simulink model "sumulacionTpBolita"  (R2019b)
settings: Solver=ode4  StartTime=0.0  StopTime=5  FixedStep=10e-6  RelTol=1e-3
undefined symbols (not defined in the file or in its folder): A0, Acd, Aoc, B0, Bcd, Boc, c, C0, Ccd, Coc, Dcd, DiscIntNeverNeededParam, Doc, K, Ki, L, Pade, Tsample, u0, x0, x0f
libraries: cstblocks x2
settings Model: Creator=mpier  LastModifiedBy=mpier
settings ConfigComp: PLC_TargetIDE=codesys23

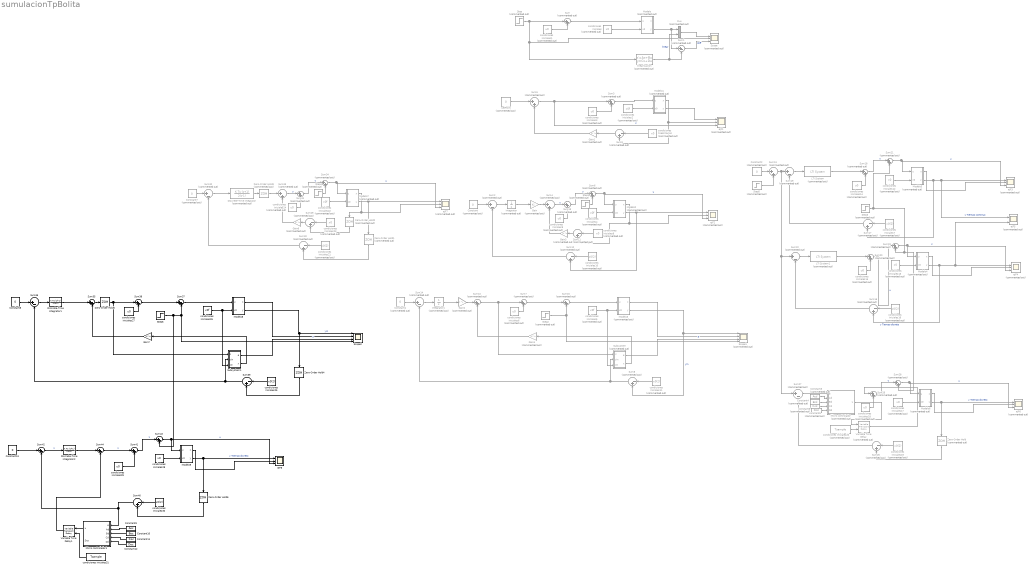
== system sumulacionTpBolita ==
  " Micro controlador" : MATLAB Function  Commented=on  TreatAsAtomicUnit=on  SystemSampleTime=Tsample
  " Micro controlador1" : MATLAB Function  TreatAsAtomicUnit=on  SystemSampleTime=Tsample
  Constant{,1..2,7} (4 alike) : Constant  Commented=on  Value=0
  Constant10 : Constant  Value=Boc
  Constant11 : Constant  Value=Coc
  Constant12 : Constant  Value=Doc
  Constant13 : Constant  Value=0
  Constant3 : Constant  Commented=on  Value=Acd
  Constant4 : Constant  Commented=on  Value=Bcd
  Constant5 : Constant  Commented=on  Value=Ccd
  Constant6 : Constant  Commented=on  Value=Dcd
  Constant8 : Constant  Value=0
  Constant9 : Constant  Value=Aoc
  Discrete-Time Integrator : DiscreteIntegrator  Commented=on  IntegratorMethod=Integration: Trapezoidal  gainval=Ki  SampleTime=Tsample  ICPrevOutput=DiscIntNeverNeededParam  ICPrevScaledInput=DiscIntNeverNeededParam
  Discrete-Time Integrator1 : DiscreteIntegrator  IntegratorMethod=Integration: Trapezoidal  gainval=Ki  SampleTime=Tsample  ICPrevOutput=DiscIntNeverNeededParam  ICPrevScaledInput=DiscIntNeverNeededParam
  Discrete-Time Integrator2 : DiscreteIntegrator  IntegratorMethod=Integration: Trapezoidal  gainval=Ki  SampleTime=Tsample  ICPrevOutput=DiscIntNeverNeededParam  ICPrevScaledInput=DiscIntNeverNeededParam
  Gain : Gain  Commented=on  Gain=Ki
  Gain{1,3..4,6} (4 alike) : Gain  Commented=on  Gain=-K  Multiplication=Matrix(K*u)
  Gain2 : Gain  Commented=on  Gain=Ki  Multiplication=Matrix(K*u)
  Gain7 : Gain  Gain=-K  Multiplication=Matrix(K*u)
  Integrator : Integrator  Commented=on
  Integrator1 : Integrator  Commented=on
  LTI System : cstblocks/LTI System  Commented=on  sys=c*Pade  IC=[]
  LTI System1 : cstblocks/LTI System  Commented=on  sys=Cd  IC=[]
  Modelo : Subsystem  Commented=on
  Modelo1 : Subsystem  Commented=on
  Modelo2 : Subsystem  Commented=on
  Modelo3 : Subsystem  Commented=on
  Modelo4 : Subsystem  Commented=on
  Modelo5 : Subsystem  Commented=on
  Modelo6 : Subsystem  Commented=on
  Modelo7 : Subsystem  Commented=on
  Modelo8 : Subsystem
  Modelo9 : Subsystem
  Mux : Mux  Commented=on  Inputs=2
  Scope : Scope  Commented=on  NumInputPorts=3
  Scope1 : Scope  Commented=on  NumInputPorts=4
  Scope2 : Scope  NumInputPorts=4
  Step : Step  Commented=on  Time=50e-3  After=0.1  SampleTime=0
  Step1 : Step  Commented=on  Time=2.5  After=10  SampleTime=0
  Step2 : Step  Commented=on  Time=2.5  After=2  SampleTime=0
  Step3 : Step  Commented=on  Time=2.5  After=100e-3  SampleTime=0
  Step4 : Step  Commented=on  Time=2.5  After=10  SampleTime=0
  Step5 : Step  Commented=on  After=1e-3  SampleTime=0
  Step6 : Step  Time=2.5  After=1e-3  SampleTime=0
  Subsystem : Subsystem  Commented=on
  Subsystem1 : Subsystem
  Sum{,3,6..7,10,13,15,18,20..21,23,26,28,31,34} (15 alike) : Sum  Commented=on  Inputs=|++
  Sum1 : Sum  Commented=on  Inputs=|+-
  Sum{8..9,11..12,16..17,25,29..30} (9 alike) : Sum  Commented=on  Inputs=|-+  OutDataTypeStr=double
  Sum{2,14,19,22,27,32} (6 alike) : Sum  Commented=on  Inputs=|+-  OutDataTypeStr=double
  Sum{4..5,24,33} (4 alike) : Sum  Commented=on  Inputs=|++  OutDataTypeStr=double
  Sum{35,37..38,41,43} (5 alike) : Sum  Inputs=|++
  Sum36 : Sum  Inputs=|+-  OutDataTypeStr=double
  Sum39 : Sum  Inputs=|-+  OutDataTypeStr=double
  Sum40 : Sum  Inputs=|-+  OutDataTypeStr=double
  Sum42 : Sum  Inputs=|+-
  Sum44 : Sum  Inputs=|+-
  Variable Time Delay : VariableTransportDelay  Commented=on  MaximumDelay=10
  Variable Time Delay1 : VariableTransportDelay  MaximumDelay=10
  Zero-Order Hold : ZeroOrderHold  Commented=on  SampleTime=Tsample
  Zero-Order Hold1 : ZeroOrderHold  Commented=on  SampleTime=-1
  Zero-Order Hold2 : ZeroOrderHold  Commented=on  SampleTime=-1
  Zero-Order Hold3 : ZeroOrderHold  Commented=on  SampleTime=-1
  Zero-Order Hold4 : ZeroOrderHold  SampleTime=-1
  Zero-Order Hold5 : ZeroOrderHold  SampleTime=-1
  Zero-Order Hold6 : ZeroOrderHold  SampleTime=Tsample
  condiciones Iniciales{,8,12..13,17,23} (6 alike) : Constant  Commented=on  Value=x0
  condiciones Iniciales{1,3,6,9,14..15,18,24} (8 alike) : Constant  Commented=on  Value=u0
  condiciones Iniciales{7,10..11,16,19,21} (6 alike) : Constant  Commented=on  Value=x0(2)
  condiciones Iniciales{2,4..5,22} (4 alike) : Constant  Commented=on  Value=x0f
  condiciones Iniciales20 : Constant  Commented=on  Value=Tsample
  condiciones Iniciales25 : Constant  Value=x0(2)
  condiciones Iniciales26 : Constant  Value=x0f
  condiciones Iniciales27 : Constant  Value=u0
  condiciones Iniciales28 : Constant  Value=x0
  condiciones Iniciales29 : Constant  Value=u0
  condiciones Iniciales30 : Constant  Value=x0(2)
  condiciones Iniciales31 : Constant  Value=Tsample
  condiciones linealizacion : Constant  Commented=on  Value=x0
  ejF{1..4,6..7} (6 alike) : Scope  Commented=on  NumInputPorts=3
  ejF5 : Scope  Commented=on  NumInputPorts=2
  ejF8 : Scope  NumInputPorts=3
  linearizacion : StateSpace  Commented=on  A=A0  B=B0  C=C0  D=0  InitialCondition=0
  setPoint : Constant  Commented=on  Value=0
  wires:
  condiciones Iniciales/1 -> Modelo/2(x0)
  Sum/1 -> Modelo/1(u)
  condiciones Iniciales1/1 -> Sum/2
  Mux/1 -> Scope/1
  Modelo/2(y) -> Sum1/1, Mux/1
  linearizacion/1 -> Sum1/2, Mux/2  "linear"
  Sum1/1 -> Scope/3  "Diff"
  Step/1 -> linearizacion/1, Scope/2, Sum/1
  Modelo1/1(x) -> Sum9/2, ejF1/2
  condiciones Iniciales3/1 -> Sum3/2
  Sum3/1 -> Modelo1/1(u)
  condiciones Iniciales2/1 -> Modelo1/2(x0)
  Modelo1/2(y) -> ejF1/1
  Sum5/1 -> ejF1/3, Sum3/1  "u"
  Gain1/1 -> Sum5/2
  Modelo2/1(x) -> ejF2/2, Sum11/2
  condiciones Iniciales4/1 -> Modelo2/2(x0)
  Constant/1 -> Sum2/1
  Sum2/1 -> Integrator/1
  Integrator/1 -> Gain/1
  Gain/1 -> Sum4/1
  condiciones Iniciales5/1 -> Subsystem/3(x0), Modelo3/2(x0)
  Sum10/1 -> Sum7/1, Subsystem/1(u)
  Gain4/1 -> Sum10/2
  Sum9/1 -> Gain1/1
  condiciones linealizacion/1 -> Sum9/1
  setPoint/1 -> Sum5/1
  Sum11/1 -> Gain3/1
  condiciones Iniciales8/1 -> Sum11/1
  Gain3/1 -> Sum4/2
  Sum12/1 -> Sum2/2
  condiciones Iniciales9/1 -> Sum13/2
  Sum4/1 -> Sum13/1  "u"
  condiciones Iniciales10/1 -> Sum12/1
  condiciones Iniciales11/1 -> Sum8/1
  Subsystem/2(x) -> Gain4/1
  condiciones Iniciales6/1 -> Sum7/2
  Sum8/1 -> Sum14/2, Subsystem/2(yin)
  Gain2/1 -> Sum10/1
  Integrator1/1 -> Gain2/1
  Constant1/1 -> Sum14/1
  Sum14/1 -> Integrator1/1
  Modelo3/2(y) -> Sum8/2, Scope1/1  "yin"
  Modelo3/1(x) -> Scope1/2
  Subsystem/1(e) -> Scope1/3  "e"
  Modelo2/2(y) -> ejF2/1, Sum12/2
  Step1/1 -> Sum6/2
  Sum13/1 -> Sum6/1  "u"
  Sum6/1 -> ejF2/3, Modelo2/1(u)  "u"
  Sum7/1 -> Sum15/1
  Step2/1 -> Sum15/2, Scope1/4
  Sum15/1 -> Modelo3/1(u)
  condiciones Iniciales14/1 -> Sum18/2
  Modelo5/2(y) -> ejF5/1, ejF3/1, Sum17/2  "y Tiempo continuo"
  Sum19/1 -> LTI System/1
  Sum18/1 -> Sum21/1  "u"
  Sum17/1 -> Sum19/2
  Modelo5/1(x) -> ejF3/2
  Sum21/1 -> ejF3/3, Modelo5/1(u)  "u"
  condiciones Iniciales7/1 -> Sum17/1
  condiciones Iniciales12/1 -> Modelo5/2(x0)
  LTI System/1 -> Sum18/1
  condiciones Iniciales16/1 -> Sum16/1
  Sum23/1 -> ejF4/3, Modelo4/1(u)  "u"
  Sum16/1 -> Sum22/2
  Sum20/1 -> Sum23/1  "u"
  Modelo4/1(x) -> ejF4/2
  Sum22/1 -> LTI System1/1
  condiciones Iniciales15/1 -> Sum20/2
  Modelo4/2(y) -> ejF5/2, ejF4/1, Sum16/2  "y Tiempo dicreto"
  condiciones Iniciales13/1 -> Modelo4/2(x0)
  LTI System1/1 -> Sum20/1
  Constant2/1 -> Sum24/1
  Step5/1 -> Sum24/2
  Step3/1 -> Sum28/2, Sum23/2, Sum21/2
  condiciones Iniciales19/1 -> Sum25/1
  condiciones Iniciales18/1 -> Sum26/2
  Sum27/1 -> " Micro controlador"/1(e)
  Sum24/1 -> Sum19/1, Sum27/1, Sum22/1
  Sum28/1 -> ejF6/3, Modelo6/1(u)  "u"
  Sum26/1 -> Sum28/1  "u"
  Modelo6/1(x) -> ejF6/2
  condiciones Iniciales17/1 -> Modelo6/2(x0)
  Modelo6/2(y) -> ejF6/1, Zero-Order Hold/1  "y Tiempo dicreto"
  Sum25/1 -> Sum27/2
  Constant3/1 -> " Micro controlador"/2(Ad)
  Constant4/1 -> " Micro controlador"/3(Bd)
  Constant5/1 -> " Micro controlador"/4(Cd)
  Constant6/1 -> " Micro controlador"/5(Dd)
  " Micro controlador"/1(u) -> Variable Time Delay/1
  Variable Time Delay/1 -> Sum26/1
  condiciones Iniciales20/1 -> Variable Time Delay/2
  Zero-Order Hold/1 -> Sum25/2
  Modelo7/1(x) -> ejF7/2, Zero-Order Hold2/1
  Sum33/1 -> Sum31/1  "u"
  condiciones Iniciales23/1 -> Sum29/1
  Sum31/1 -> Sum34/1  "u"
  Modelo7/2(y) -> ejF7/1, Zero-Order Hold1/1
  Gain6/1 -> Sum33/2
  Sum32/1 -> Discrete-Time Integrator/1
  Step4/1 -> Sum34/2
  Discrete-Time Integrator/1 -> Zero-Order Hold3/1
  Sum34/1 -> ejF7/3, Modelo7/1(u)  "u"
  condiciones Iniciales21/1 -> Sum30/1
  Sum30/1 -> Sum32/2
  Sum29/1 -> Gain6/1
  condiciones Iniciales24/1 -> Sum31/2
  condiciones Iniciales22/1 -> Modelo7/2(x0)
  Constant7/1 -> Sum32/1
  Zero-Order Hold1/1 -> Sum30/2
  Zero-Order Hold2/1 -> Sum29/2
  Zero-Order Hold3/1 -> Sum33/1
  Sum36/1 -> Discrete-Time Integrator1/1
  Modelo8/2(y) -> Zero-Order Hold4/1, Scope2/1  "yin"
  Sum37/1 -> Modelo8/1(u)
  Modelo8/1(x) -> Scope2/2
  Sum35/1 -> Zero-Order Hold5/1
  condiciones Iniciales25/1 -> Sum39/1
  Sum38/1 -> Sum37/1
  Subsystem1/2(x) -> Gain7/1
  condiciones Iniciales27/1 -> Sum38/2
  condiciones Iniciales26/1 -> Subsystem1/3(x0), Modelo8/2(x0)
  Gain7/1 -> Sum35/2
  Discrete-Time Integrator1/1 -> Sum35/1
  Subsystem1/1(e) -> Scope2/3  "e"
  Sum39/1 -> Sum36/2, Subsystem1/2(yin)
  Zero-Order Hold4/1 -> Sum39/2
  Zero-Order Hold5/1 -> Subsystem1/1(u), Sum38/1
  condiciones Iniciales31/1 -> Variable Time Delay1/2
  Constant11/1 -> " Micro controlador1"/4(Cd)
  Constant10/1 -> " Micro controlador1"/3(Bd)
  condiciones Iniciales29/1 -> Sum41/2
  Sum43/1 -> ejF8/3, Modelo9/1(u)  "u"
  Modelo9/1(x) -> ejF8/2
  Zero-Order Hold6/1 -> Sum40/2
  Sum41/1 -> Sum43/1  "u"
  Constant12/1 -> " Micro controlador1"/5(Dd)
  Constant9/1 -> " Micro controlador1"/2(Ad)
  condiciones Iniciales28/1 -> Modelo9/2(x0)
  Constant8/1 -> Sum36/1
  condiciones Iniciales30/1 -> Sum40/1
  Step6/1 -> Sum43/2, Sum37/2, Scope2/4
  Modelo9/2(y) -> ejF8/1, Zero-Order Hold6/1  "y Tiempo dicreto"
  " Micro controlador1"/1(u) -> Variable Time Delay1/1
  Sum42/1 -> Discrete-Time Integrator2/1  "u"
  Sum40/1 -> Sum42/2, " Micro controlador1"/1(e)
  Sum44/1 -> Sum41/1  "u"
  Discrete-Time Integrator2/1 -> Sum44/1
  Variable Time Delay1/1 -> Sum44/2
  Constant13/1 -> Sum42/1

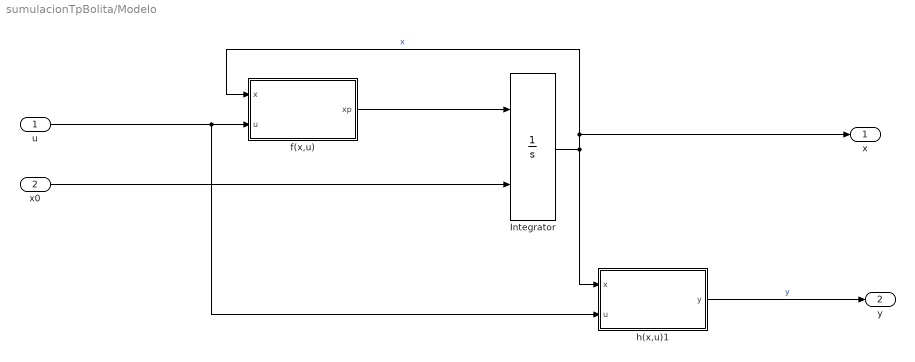
== system sumulacionTpBolita/Modelo ==
  u : Inport
  x0 : Inport  Port=2
  Integrator : Integrator  InitialConditionSource=external
  f(x,u) : MATLAB Function  TreatAsAtomicUnit=on
  h(x,u)1 : MATLAB Function  TreatAsAtomicUnit=on
  x : Outport
  y : Outport  Port=2
  wires:
  Integrator/1 -> x/1, f(x,u)/1(x), h(x,u)1/1(x)  "x"
  f(x,u)/1(xp) -> Integrator/1
  x0/1 -> Integrator/2
  u/1 -> h(x,u)1/2(u), f(x,u)/2(u)
  h(x,u)1/1(y) -> y/1  "y"

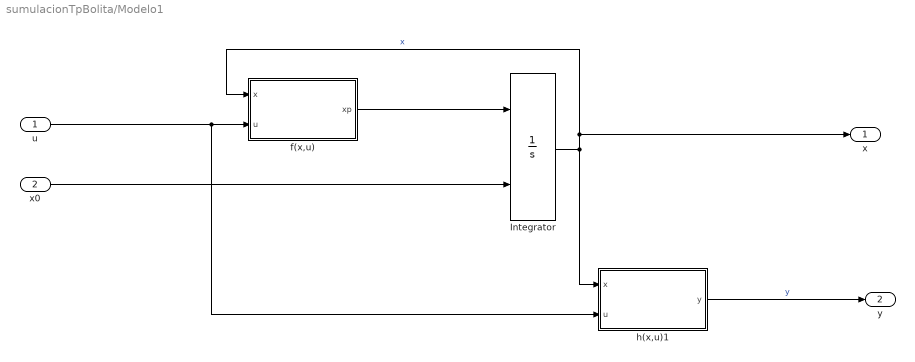
== system sumulacionTpBolita/Modelo1 ==
  u : Inport
  x0 : Inport  Port=2
  Integrator : Integrator  InitialConditionSource=external
  f(x,u) : MATLAB Function  TreatAsAtomicUnit=on
  h(x,u)1 : MATLAB Function  TreatAsAtomicUnit=on
  x : Outport
  y : Outport  Port=2
  wires:
  Integrator/1 -> x/1, f(x,u)/1(x), h(x,u)1/1(x)  "x"
  f(x,u)/1(xp) -> Integrator/1
  x0/1 -> Integrator/2
  u/1 -> h(x,u)1/2(u), f(x,u)/2(u)
  h(x,u)1/1(y) -> y/1  "y"

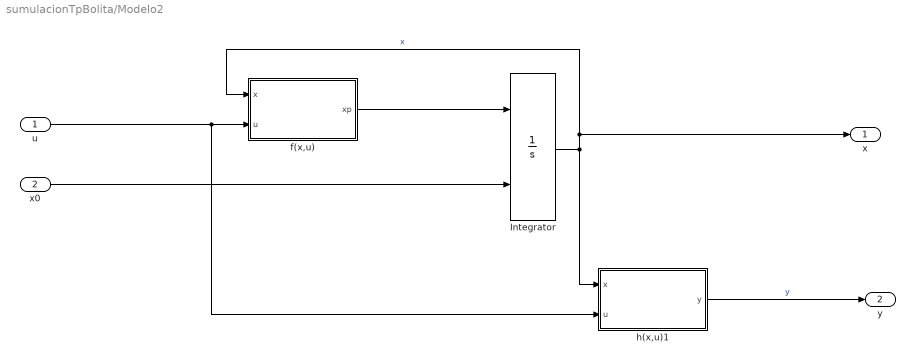
== system sumulacionTpBolita/Modelo2 ==
  u : Inport
  x0 : Inport  Port=2
  Integrator : Integrator  InitialConditionSource=external
  f(x,u) : MATLAB Function  TreatAsAtomicUnit=on
  h(x,u)1 : MATLAB Function  TreatAsAtomicUnit=on
  x : Outport
  y : Outport  Port=2
  wires:
  Integrator/1 -> x/1, f(x,u)/1(x), h(x,u)1/1(x)  "x"
  f(x,u)/1(xp) -> Integrator/1
  x0/1 -> Integrator/2
  u/1 -> h(x,u)1/2(u), f(x,u)/2(u)
  h(x,u)1/1(y) -> y/1  "y"

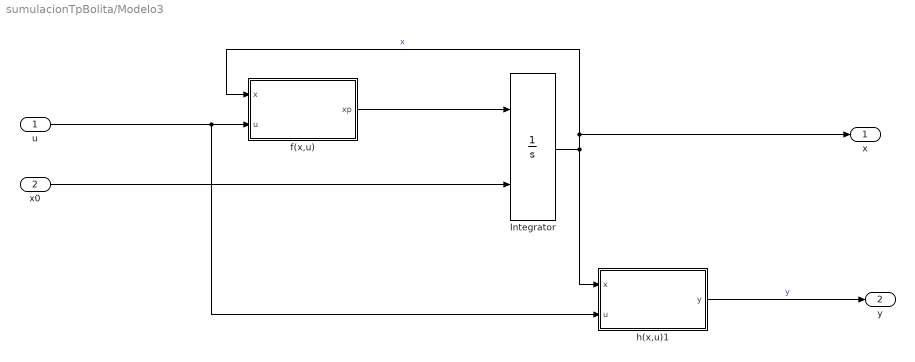
== system sumulacionTpBolita/Modelo3 ==
  u : Inport
  x0 : Inport  Port=2
  Integrator : Integrator  InitialConditionSource=external
  f(x,u) : MATLAB Function  TreatAsAtomicUnit=on
  h(x,u)1 : MATLAB Function  TreatAsAtomicUnit=on
  x : Outport
  y : Outport  Port=2
  wires:
  Integrator/1 -> x/1, f(x,u)/1(x), h(x,u)1/1(x)  "x"
  f(x,u)/1(xp) -> Integrator/1
  x0/1 -> Integrator/2
  u/1 -> h(x,u)1/2(u), f(x,u)/2(u)
  h(x,u)1/1(y) -> y/1  "y"

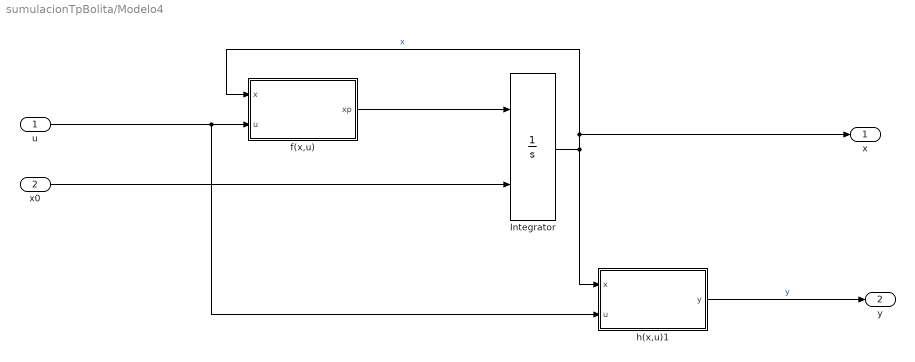
== system sumulacionTpBolita/Modelo4 ==
  u : Inport
  x0 : Inport  Port=2
  Integrator : Integrator  InitialConditionSource=external
  f(x,u) : MATLAB Function  TreatAsAtomicUnit=on
  h(x,u)1 : MATLAB Function  TreatAsAtomicUnit=on
  x : Outport
  y : Outport  Port=2
  wires:
  Integrator/1 -> x/1, f(x,u)/1(x), h(x,u)1/1(x)  "x"
  f(x,u)/1(xp) -> Integrator/1
  x0/1 -> Integrator/2
  u/1 -> h(x,u)1/2(u), f(x,u)/2(u)
  h(x,u)1/1(y) -> y/1  "y"

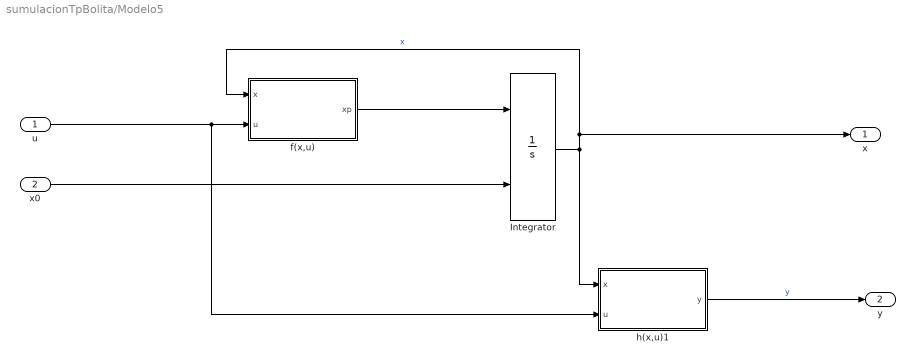
== system sumulacionTpBolita/Modelo5 ==
  u : Inport
  x0 : Inport  Port=2
  Integrator : Integrator  InitialConditionSource=external
  f(x,u) : MATLAB Function  TreatAsAtomicUnit=on
  h(x,u)1 : MATLAB Function  TreatAsAtomicUnit=on
  x : Outport
  y : Outport  Port=2
  wires:
  Integrator/1 -> x/1, f(x,u)/1(x), h(x,u)1/1(x)  "x"
  f(x,u)/1(xp) -> Integrator/1
  x0/1 -> Integrator/2
  u/1 -> h(x,u)1/2(u), f(x,u)/2(u)
  h(x,u)1/1(y) -> y/1  "y"

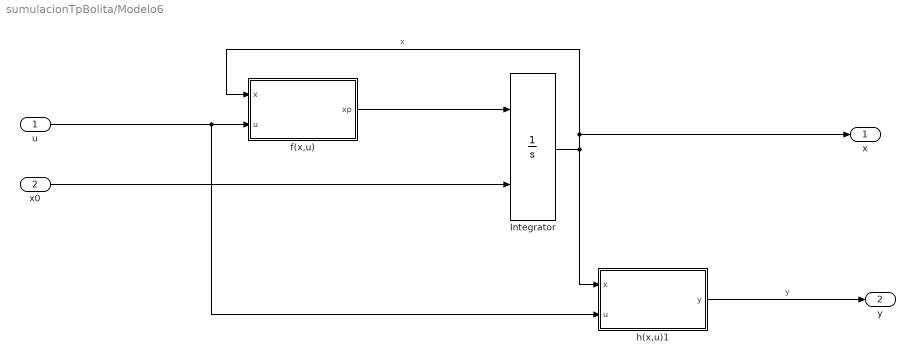
== system sumulacionTpBolita/Modelo6 ==
  u : Inport
  x0 : Inport  Port=2
  Integrator : Integrator  InitialConditionSource=external
  f(x,u) : MATLAB Function  TreatAsAtomicUnit=on
  h(x,u)1 : MATLAB Function  TreatAsAtomicUnit=on
  x : Outport
  y : Outport  Port=2
  wires:
  Integrator/1 -> x/1, f(x,u)/1(x), h(x,u)1/1(x)  "x"
  f(x,u)/1(xp) -> Integrator/1
  x0/1 -> Integrator/2
  u/1 -> h(x,u)1/2(u), f(x,u)/2(u)
  h(x,u)1/1(y) -> y/1  "y"

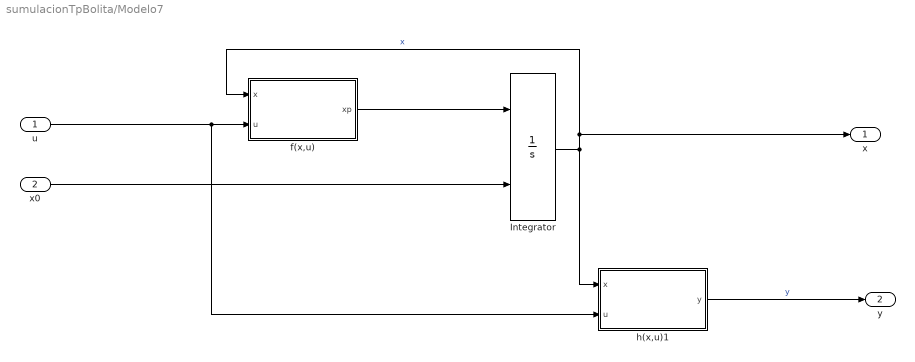
== system sumulacionTpBolita/Modelo7 ==
  u : Inport
  x0 : Inport  Port=2
  Integrator : Integrator  InitialConditionSource=external
  f(x,u) : MATLAB Function  TreatAsAtomicUnit=on
  h(x,u)1 : MATLAB Function  TreatAsAtomicUnit=on
  x : Outport
  y : Outport  Port=2
  wires:
  Integrator/1 -> x/1, f(x,u)/1(x), h(x,u)1/1(x)  "x"
  f(x,u)/1(xp) -> Integrator/1
  x0/1 -> Integrator/2
  u/1 -> h(x,u)1/2(u), f(x,u)/2(u)
  h(x,u)1/1(y) -> y/1  "y"

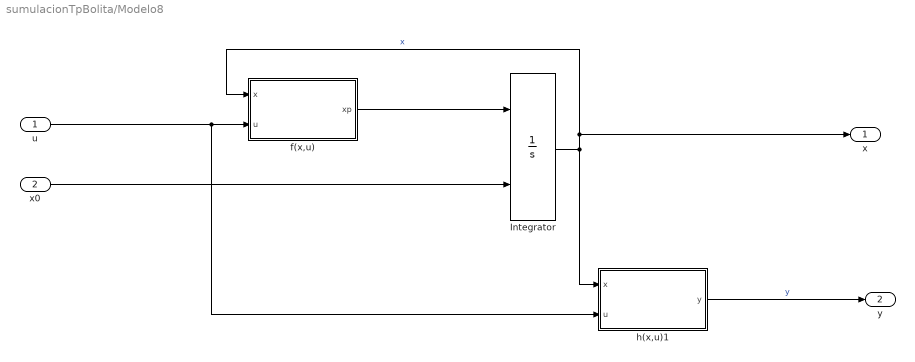
== system sumulacionTpBolita/Modelo8 ==
  u : Inport
  x0 : Inport  Port=2
  Integrator : Integrator  InitialConditionSource=external
  f(x,u) : MATLAB Function  TreatAsAtomicUnit=on
  h(x,u)1 : MATLAB Function  TreatAsAtomicUnit=on
  x : Outport
  y : Outport  Port=2
  wires:
  Integrator/1 -> x/1, f(x,u)/1(x), h(x,u)1/1(x)  "x"
  f(x,u)/1(xp) -> Integrator/1
  x0/1 -> Integrator/2
  u/1 -> h(x,u)1/2(u), f(x,u)/2(u)
  h(x,u)1/1(y) -> y/1  "y"

== system sumulacionTpBolita/Modelo9 ==
  u : Inport
  x0 : Inport  Port=2
  Integrator : Integrator  InitialConditionSource=external
  f(x,u) : MATLAB Function  TreatAsAtomicUnit=on
  h(x,u)1 : MATLAB Function  TreatAsAtomicUnit=on
  x : Outport
  y : Outport  Port=2
  wires:
  Integrator/1 -> x/1, f(x,u)/1(x), h(x,u)1/1(x)  "x"
  f(x,u)/1(xp) -> Integrator/1
  x0/1 -> Integrator/2
  u/1 -> h(x,u)1/2(u), f(x,u)/2(u)
  h(x,u)1/1(y) -> y/1  "y"

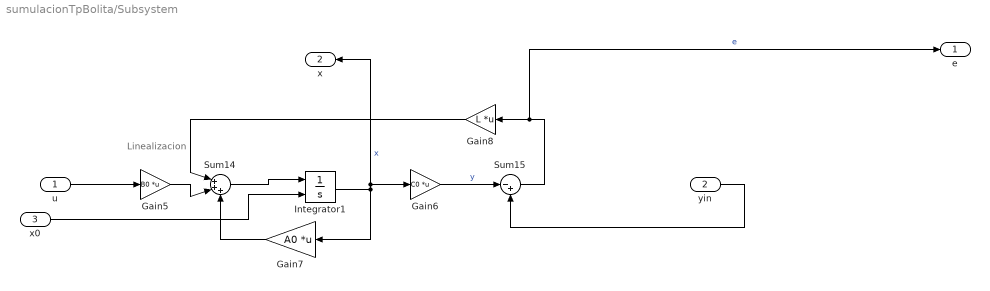
== system sumulacionTpBolita/Subsystem ==
  note: Linealizacion
  u : Inport
  yin : Inport  Port=2
  x0 : Inport  Port=3
  Gain5 : Gain  Gain=B0  Multiplication=Matrix(K*u)
  Gain6 : Gain  Gain=C0  Multiplication=Matrix(K*u)
  Gain7 : Gain  Gain=A0  Multiplication=Matrix(K*u)
  Gain8 : Gain  Gain=L  Multiplication=Matrix(K*u)
  Integrator1 : Integrator  InitialConditionSource=external
  Sum14 : Sum  Inputs=|+++
  Sum15 : Sum  Inputs=|-+
  e : Outport
  x : Outport  Port=2
  wires:
  u/1 -> Gain5/1
  Sum14/1 -> Integrator1/1
  yin/1 -> Sum15/2
  Integrator1/1 -> x/1, Gain6/1, Gain7/1  "x"
  Gain7/1 -> Sum14/3
  Sum15/1 -> e/1, Gain8/1  "e"
  Gain6/1 -> Sum15/1  "y"
  Gain5/1 -> Sum14/2
  Gain8/1 -> Sum14/1
  x0/1 -> Integrator1/2

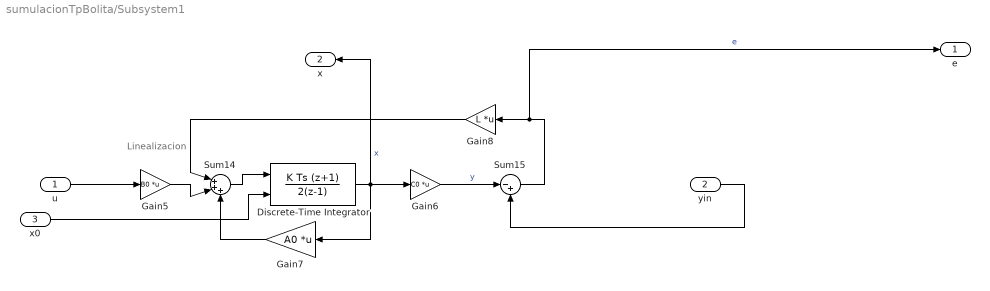
== system sumulacionTpBolita/Subsystem1 ==
  note: Linealizacion
  u : Inport
  yin : Inport  Port=2
  x0 : Inport  Port=3
  Discrete-Time Integrator : DiscreteIntegrator  IntegratorMethod=Integration: Trapezoidal  InitialConditionSource=external  SampleTime=Tsample  ICPrevOutput=DiscIntNeverNeededParam  ICPrevScaledInput=DiscIntNeverNeededParam
  Gain5 : Gain  Gain=B0  Multiplication=Matrix(K*u)
  Gain6 : Gain  Gain=C0  Multiplication=Matrix(K*u)
  Gain7 : Gain  Gain=A0  Multiplication=Matrix(K*u)
  Gain8 : Gain  Gain=L  Multiplication=Matrix(K*u)
  Sum14 : Sum  Inputs=|+++
  Sum15 : Sum  Inputs=|-+
  e : Outport
  x : Outport  Port=2
  wires:
  u/1 -> Gain5/1
  Sum14/1 -> Discrete-Time Integrator/1
  yin/1 -> Sum15/2
  Discrete-Time Integrator/1 -> x/1, Gain7/1, Gain6/1  "x"
  Gain7/1 -> Sum14/3
  Sum15/1 -> e/1, Gain8/1  "e"
  Gain6/1 -> Sum15/1  "y"
  Gain5/1 -> Sum14/2
  Gain8/1 -> Sum14/1
  x0/1 -> Discrete-Time Integrator/2

== matlab function sumulacionTpBolita/Modelo/h(x,u)1 ==
  data: x input; u input; y output
function y = h(x,u)



y=x(2);

== matlab function sumulacionTpBolita/Modelo/f(x,u) ==
  data: x input; u input; xp output
function xp = f(x,u)



R=4;%resistencia del inductor
 L=1;%inductancia del electro iman
 m=0.2;%masa de la bolita
 g=10;%aceleracion de la grabedad
 

ids=(-(x(1)^2)/(L/R))+(u/L);

F1s=(0.5*((2+x(1))^2))/((1-x(2))^2);
F2s=(0.5*((2-x(1))^2))/((1+x(2))^2);
vds=-g+(F1s/m)-(F2s/m);

xp=[ids;x(3);vds];

== matlab function sumulacionTpBolita/Modelo1/f(x,u) ==
  data: x input; u input; xp output
function xp = f(x,u)



R=4;%resistencia del inductor
 L=1;%inductancia del electro iman
 m=0.2;%masa de la bolita
 g=10;%aceleracion de la grabedad
 

ids=(-(x(1)^2)/(L/R))+(u/L);

F1s=(0.5*((2+x(1))^2))/((1-x(2))^2);
F2s=(0.5*((2-x(1))^2))/((1+x(2))^2);
vds=-g+(F1s/m)-(F2s/m);

xp=[ids;x(3);vds];

== matlab function sumulacionTpBolita/Modelo1/h(x,u)1 ==
  data: x input; u input; y output
function y = h(x,u)



y=x(2);

== matlab function sumulacionTpBolita/Modelo2/f(x,u) ==
  data: x input; u input; xp output
function xp = f(x,u)



R=4;%resistencia del inductor
 L=1;%inductancia del electro iman
 m=0.2;%masa de la bolita
 g=10;%aceleracion de la grabedad
 

ids=(-(x(1)^2)/(L/R))+(u/L);

F1s=(0.5*((2+x(1))^2))/((1-x(2))^2);
F2s=(0.5*((2-x(1))^2))/((1+x(2))^2);
vds=-g+(F1s/m)-(F2s/m);

xp=[ids;x(3);vds];

== matlab function sumulacionTpBolita/Modelo2/h(x,u)1 ==
  data: x input; u input; y output
function y = h(x,u)



y=x(2);

== matlab function sumulacionTpBolita/Modelo3/f(x,u) ==
  data: x input; u input; xp output
function xp = f(x,u)



R=4;%resistencia del inductor
 L=1;%inductancia del electro iman
 m=0.2;%masa de la bolita
 g=10;%aceleracion de la grabedad
 

ids=(-(x(1)^2)/(L/R))+(u/L);

F1s=(0.5*((2+x(1))^2))/((1-x(2))^2);
F2s=(0.5*((2-x(1))^2))/((1+x(2))^2);
vds=-g+(F1s/m)-(F2s/m);

xp=[ids;x(3);vds];

== matlab function sumulacionTpBolita/Modelo3/h(x,u)1 ==
  data: x input; u input; y output
function y = h(x,u)



y=x(2);

== matlab function sumulacionTpBolita/Modelo4/f(x,u) ==
  data: x input; u input; xp output
function xp = f(x,u)



R=4;%resistencia del inductor
 L=1;%inductancia del electro iman
 m=0.2;%masa de la bolita
 g=10;%aceleracion de la grabedad
 

ids=(-(x(1)^2)/(L/R))+(u/L);

F1s=(0.5*((2+x(1))^2))/((1-x(2))^2);
F2s=(0.5*((2-x(1))^2))/((1+x(2))^2);
vds=-g+(F1s/m)-(F2s/m);

xp=[ids;x(3);vds];

== matlab function sumulacionTpBolita/Modelo4/h(x,u)1 ==
  data: x input; u input; y output
function y = h(x,u)



y=x(2);

== matlab function sumulacionTpBolita/Modelo5/f(x,u) ==
  data: x input; u input; xp output
function xp = f(x,u)



R=4;%resistencia del inductor
 L=1;%inductancia del electro iman
 m=0.2;%masa de la bolita
 g=10;%aceleracion de la grabedad
 

ids=(-(x(1)^2)/(L/R))+(u/L);

F1s=(0.5*((2+x(1))^2))/((1-x(2))^2);
F2s=(0.5*((2-x(1))^2))/((1+x(2))^2);
vds=-g+(F1s/m)-(F2s/m);

xp=[ids;x(3);vds];

== matlab function sumulacionTpBolita/Modelo5/h(x,u)1 ==
  data: x input; u input; y output
function y = h(x,u)



y=x(2);

== matlab function sumulacionTpBolita/ Micro controlador ==
  data: e input; u output; Ad input; Bd input; Cd input; Dd input
function u = fcn(e,Ad,Bd,Cd,Dd)

persistent xp;

if isempty(xp)
    xp =[0;0;0;0];
end
xp1=[0;0;0;0];
xp1=Ad*xp+Bd*e;
u=transpose(Cd)*xp+Dd*e;

xp=xp1;
end

== matlab function sumulacionTpBolita/Modelo6/f(x,u) ==
  data: x input; u input; xp output
function xp = f(x,u)



R=4;%resistencia del inductor
 L=1;%inductancia del electro iman
 m=0.2;%masa de la bolita
 g=10;%aceleracion de la grabedad
 

ids=(-(x(1)^2)/(L/R))+(u/L);

F1s=(0.5*((2+x(1))^2))/((1-x(2))^2);
F2s=(0.5*((2-x(1))^2))/((1+x(2))^2);
vds=-g+(F1s/m)-(F2s/m);

xp=[ids;x(3);vds];

== matlab function sumulacionTpBolita/Modelo6/h(x,u)1 ==
  data: x input; u input; y output
function y = h(x,u)



y=x(2);

== matlab function sumulacionTpBolita/Modelo7/f(x,u) ==
  data: x input; u input; xp output
function xp = f(x,u)



R=4;%resistencia del inductor
 L=1;%inductancia del electro iman
 m=0.2;%masa de la bolita
 g=10;%aceleracion de la grabedad
 

ids=(-(x(1)^2)/(L/R))+(u/L);

F1s=(0.5*((2+x(1))^2))/((1-x(2))^2);
F2s=(0.5*((2-x(1))^2))/((1+x(2))^2);
vds=-g+(F1s/m)-(F2s/m);

xp=[ids;x(3);vds];

== matlab function sumulacionTpBolita/Modelo7/h(x,u)1 ==
  data: x input; u input; y output
function y = h(x,u)



y=x(2);

== matlab function sumulacionTpBolita/Modelo8/f(x,u) ==
  data: x input; u input; xp output
function xp = f(x,u)



R=4;%resistencia del inductor
 L=1;%inductancia del electro iman
 m=0.2;%masa de la bolita
 g=10;%aceleracion de la grabedad
 

ids=(-(x(1)^2)/(L/R))+(u/L);

F1s=(0.5*((2+x(1))^2))/((1-x(2))^2);
F2s=(0.5*((2-x(1))^2))/((1+x(2))^2);
vds=-g+(F1s/m)-(F2s/m);

xp=[ids;x(3);vds];

== matlab function sumulacionTpBolita/Modelo8/h(x,u)1 ==
  data: x input; u input; y output
function y = h(x,u)



y=x(2);

== matlab function sumulacionTpBolita/ Micro controlador1 ==
  data: e input; u output; Ad input; Bd input; Cd input; Dd input; Sxp output
function [u,Sxp] = fcn( e,Ad,Bd,Cd,Dd)

persistent xp;

if isempty(xp)
    xp =[0;0;0];
end
xp1=[0;0;0];
xp1=Ad*xp+Bd*e;
u=transpose(Cd)*xp+Dd*e;

xp=xp1;
Sxp=xp;
end

== matlab function sumulacionTpBolita/Modelo9/f(x,u) ==
  data: x input; u input; xp output
function xp = f(x,u)



R=4;%resistencia del inductor
 L=1;%inductancia del electro iman
 m=0.2;%masa de la bolita
 g=10;%aceleracion de la grabedad
 

ids=(-(x(1)^2)/(L/R))+(u/L);

F1s=(0.5*((2+x(1))^2))/((1-x(2))^2);
F2s=(0.5*((2-x(1))^2))/((1+x(2))^2);
vds=-g+(F1s/m)-(F2s/m);

xp=[ids;x(3);vds];

== matlab function sumulacionTpBolita/Modelo9/h(x,u)1 ==
  data: x input; u input; y output
function y = h(x,u)



y=x(2);
